simulink model "NN_MPC"  (R2025b)
settings: Solver=FixedStepDiscrete  StartTime=0.0  StopTime=8000  RelTol=1e-3
values from neighbouring files (symbols this model uses):
  BIAS_NN = 0    [setup_MPC_NN_simple_v5.m]
undefined symbols (not defined in the file or in its folder): dspblkCoreblockFVToolHelper, gcbh
libraries: mpclib x1
settings Model: Creator=Usuario  LastModifiedBy=Usuario

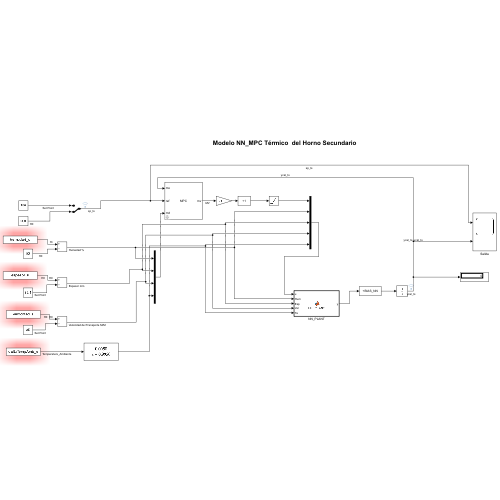
[thumbnail: Simulink's stored preview of the top-level diagram]
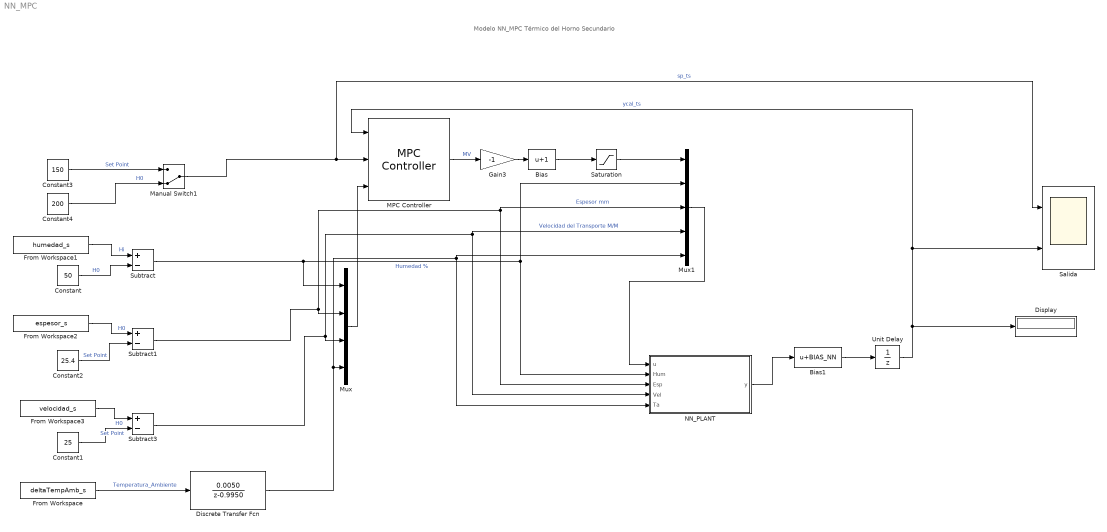
== system NN_MPC ==
  note: Modelo NN_MPC Térmico del Horno Secundario
  Bias : Bias  Bias=1  SaturateOnIntegerOverflow=off
  Bias1 : Bias  Bias=BIAS_NN  SaturateOnIntegerOverflow=off
  Constant : Constant  Value=50
  Constant1 : Constant  Value=25
  Constant2 : Constant  Value=25.4
  Constant3 : Constant  Value=150
  Constant4 : Constant  Value=200
  Discrete Transfer Fcn : DiscreteTransferFcn  LoadFcn=dspblkCoreblockFVToolHelper(gcbh,'load');  Numerator=[0 0.0050]  Denominator=[1 -0.9950]
      settings: CopyFcn=dspblkCoreblockFVToolHelper(gcbh,'copy');  DeleteFcn=dspblkCoreblockFVToolHelper(gcbh,'close');  ModelCloseFcn=dspblkCoreblockFVToolHelper(gcbh,'close');  PreSaveFcn=dspblkCoreblockFVToolHelper(gcbh,'presave');  PostSaveFcn=dspblkCoreblockFVToolHelper(gcbh,'postsave');  CloseFcn=dspblkCoreblockFVToolHelper(gcbh,'close');
  Display : Display
      settings: Decimation=2
  From Workspace : FromWorkspace  VariableName=deltaTempAmb_s  OutputAfterFinalValue=Holding final value
  From Workspace1 : FromWorkspace  VariableName=humedad_s  OutputAfterFinalValue=Holding final value
  From Workspace2 : FromWorkspace  VariableName=espesor_s  OutputAfterFinalValue=Holding final value
  From Workspace3 : FromWorkspace  VariableName=velocidad_s  OutputAfterFinalValue=Holding final value
  Gain3 : Gain  Gain=-1
  MPC Controller : mpclib/MPC Controller  SCDEnableBlockLinearizationSpecification=on  mpcobj=mpcobj_nn  is_multiple=0  enable_value=0  return_u0=off  updateMPCinCallerWorkspace=on  md_inport=on  mv_inport=off  uref_inport=off  return_cost=off  return_mvseq=off  return_qpstatus=off  return_xseq=off  return_state=off  return_ovseq=off  state_inport=off  umin_inport=off  umax_inport=off  ymin_inport=off  ymax_inport=off  cc_inport=off  ywt_inport=off  uwt_inport=off  duwt_inport=off  rhoeps_inport=off  pm_inport=off  MaximumP=10  HorizonChoice=FixedHorizon  n_ts=1  n_p=18  n_mv=1  n_md=4  n_ud=0  n_mo=1  n_uo=0  BlockDataType=double  SampleTimeInherited=off  switch_inport=off
  Manual Switch1 : ManualSwitch  CurrentSetting=0
  Mux : Mux
  Mux1 : Mux  Inputs=5
  NN_PLANT : MATLAB Function  TreatAsAtomicUnit=on
  Salida : Scope  NumInputPorts=2
      settings: ActiveDisplayYMinimum=-24.999999999999993  ActiveDisplayYMaximum=225  DataLoggingVariableName=ScopeData2
  Saturation : Saturate  UpperLimit=1  LowerLimit=0
  Subtract : Sum  Inputs=+-
  Subtract1 : Sum  Inputs=+-
  Subtract3 : Sum  Inputs=+-
  Unit Delay : UnitDelay  HasFrameUpgradeWarning=on
  wires:
  Subtract3/1 -> NN_PLANT/4(Vel), Mux1/4, Mux/3  "Velocidad del Transporte M/M"
  Constant/1 -> Subtract/2  "H0"
  Subtract/1 -> NN_PLANT/2(Hum), Mux1/2, Mux/1  "Humedad %"
  From Workspace1/1 -> Subtract/1  "Hi"
  MPC Controller/1 -> Gain3/1  "MV"
  Subtract1/1 -> NN_PLANT/3(Esp), Mux1/3, Mux/2  "Espesor mm"
  Discrete Transfer Fcn/1 -> NN_PLANT/5(Ta), Mux1/5, Mux/4
  From Workspace2/1 -> Subtract1/1  "H0"
  From Workspace3/1 -> Subtract3/1  "H0"
  Constant4/1 -> Manual Switch1/2  "H0"
  From Workspace/1 -> Discrete Transfer Fcn/1  "Temperatura_Ambiente"
  Constant1/1 -> Subtract3/2  "Set Point"
  Constant2/1 -> Subtract1/2  "Set Point"
  Mux/1 -> MPC Controller/3
  Constant3/1 -> Manual Switch1/1  "Set Point"
  Unit Delay/1 -> MPC Controller/1, Salida/2, Display/1  "ycal_ts"
  Manual Switch1/1 -> MPC Controller/2, Salida/1  "sp_ts"
  Bias1/1 -> Unit Delay/1
  Bias/1 -> Saturation/1
  Saturation/1 -> Mux1/1
  Gain3/1 -> Bias/1
  Mux1/1 -> NN_PLANT/1(u)
  NN_PLANT/1(y) -> Bias1/1

== matlab function NN_MPC/NN_PLANT ==
  data: u input; y output; Hum input; Esp input; Vel input; Ta input
function y = NN_PLANT(u, Hum, Esp, Vel, Ta)
%#codegen
% Adapter de la NN a Simulink.
% Entradas: u en pu (Saturada 0..1), Hum/Esp/Vel/Ta escalares.
% Salida: y_raw (sin bias). El bias lo aplicas fuera con +BIAS_NN.

coder.extrinsic('nn_horno_predict');

% fuerza double escalar
u   = double(u(1));
Hum = double(Hum(1));
Esp = double(Esp(1));
Vel = double(Vel(1));
Ta  = double(Ta(1));

% seguridad de rango para la red (por si llega algo fuera)
if u < 0, u = 0; end
if u > 1, u = 1; end

phi = [u; Hum; Esp; Vel; Ta];

y = 0.0;                     % prealoca tipo
tmp = nn_horno_predict(phi); % la función ya normaliza/denormaliza adentro
if ~isempty(tmp)
    y = double(tmp);
end
end
